simulink model "XYGraph"  (Simulink 8.0)
settings: Solver=ode45  StartTime=0.0  StopTime=10.0  RelTol=1e-3
libraries: simulink x2
settings Model: Creator=Faradars  LastModifiedBy=Faradars

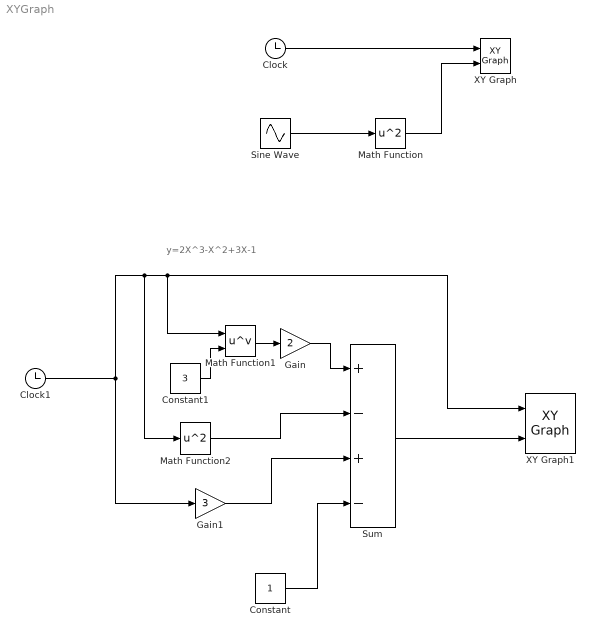
== system XYGraph ==
  note: y=2X^3-X^2+3X-1
  Clock : Clock
  Clock1 : Clock
  Constant : Constant
  Constant1 : Constant  Value=3
  Gain : Gain  Gain=2
  Gain1 : Gain  Gain=3
  Math Function : Math  Operator=square  SaturateOnIntegerOverflow=on
  Math Function1 : Math  Operator=pow  SaturateOnIntegerOverflow=on
  Math Function2 : Math  Operator=square  SaturateOnIntegerOverflow=on
  Sine Wave : Sin  SampleTime=0
  Sum : Sum  Inputs=+-+-
  XY Graph : simulink/Sinks/XY Graph  xmin=0  xmax=2*pi  ymin=-0.5  ymax=1.5  st=-1
  XY Graph1 : simulink/Sinks/XY Graph  xmin=-5  xmax=5  ymin=-150  ymax=150  st=-1
  wires:
  Sine Wave/1 -> Math Function/1
  Math Function/1 -> XY Graph/2
  Clock/1 -> XY Graph/1
  Sum/1 -> XY Graph1/2
  Clock1/1 -> Math Function2/1, XY Graph1/1, Math Function1/1, Gain1/1
  Constant/1 -> Sum/4
  Constant1/1 -> Math Function1/2
  Math Function1/1 -> Gain/1
  Gain/1 -> Sum/1
  Math Function2/1 -> Sum/2
  Gain1/1 -> Sum/3
